simulink library "flatball_6dof_plnt_lib"  (R2021b)
settings: Solver=VariableStepAuto  StartTime=0.0  StopTime=10.0  RelTol=1e-3
values from neighbouring files (symbols this model uses):
  amb = evalin( 'base', 'amb')    [flatball_6dof_eqom.m]
  C = evalin( 'base', 'C')    [flatball_6dof_eqom.m]
  disc = evalin( 'base', 'disc')    [flatball_6dof_eqom.m]    (also in flatball_6dof_init.m = struct; flatball_init_disc_params.m = struct)
  X0_z1m_at_rest = [1e-3 1e-3 -1, -1e-6 1e-6 -1e-6, 0 0 1e-6, 0 0 -1e-6]    [flatball_6dof_wrk.m]    (also in hummel_thesis_mdl_validation.m)
  Y0 = [0 0 -1, 0 15*C.DEG2RAD 0, 15 0 0, 0 0 (2*15*0.29/disc.d)]    [flatball_6dof_eqom.m]
undefined symbols (not defined in the file or in its folder): CandP, flatball
libraries: simulink x6, aerolibanim x2, aerolibnav x2, matrix_library x2, $bdroot x1, mspfiltlib x1
(part 1 of 3)
settings Model: Creator=schae  LastModifiedBy=schae

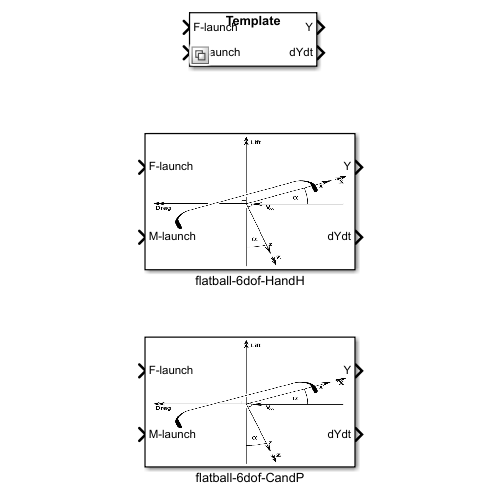
[thumbnail: Simulink's stored preview of the top-level diagram]
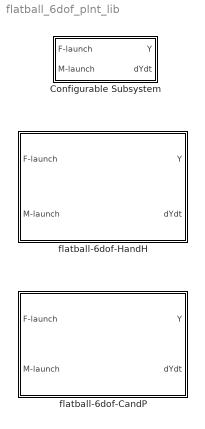
== system flatball_6dof_plnt_lib ==
  Configurable Subsystem : Subsystem  BlockChoice=flatball-6dof-CandP
      settings: TemplateBlock=self  MemberBlocks=flatball-6dof-CandP,flatball-6dof-HandH
  flatball-6dof-CandP : Subsystem
      mask Display: image('C:\.local\desktop\flatball-dev-main-misc.protolabs\media\img\screenshots\flatball-6dof.png'); % Use "Edit Image" on toolstrip to change.
  flatball-6dof-HandH : Subsystem
      mask Display: image('C:\.local\desktop\flatball-dev-main-misc.protolabs\media\img\screenshots\flatball-6dof.png'); % Use "Edit Image" on toolstrip to change.

== system flatball_6dof_plnt_lib/Configurable Subsystem ==
  F-launch : Inport
  M-launch : Inport  Port=2
  flatball-6dof-CandP : $bdroot/flatball-6dof-CandP  SystemSampleTime=-1  VariantActivationTime=update diagram  Latency=0  AutoFrameSizeCalculation=off
  Y : Outport
  dYdt : Outport  Port=2
  wires:
  F-launch/1 -> flatball-6dof-CandP/1
  M-launch/1 -> flatball-6dof-CandP/2
  flatball-6dof-CandP/1 -> Y/1
  flatball-6dof-CandP/2 -> dYdt/1

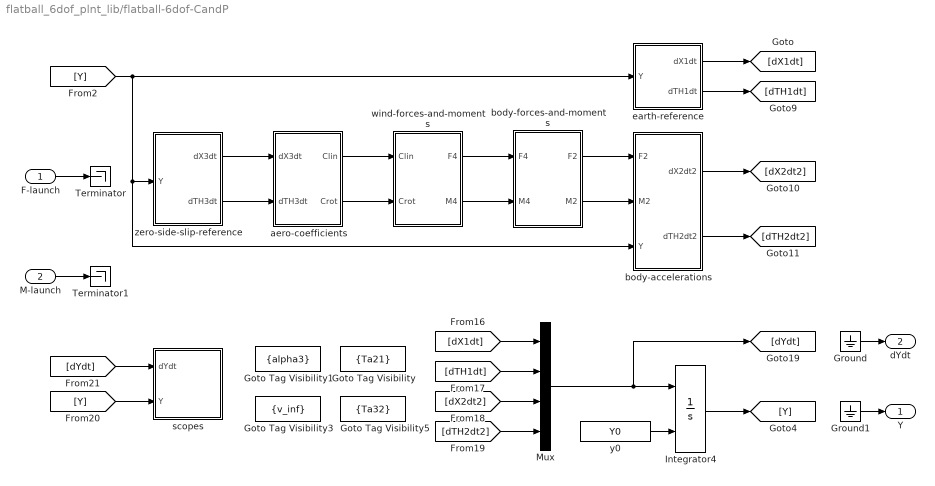
== system flatball_6dof_plnt_lib/flatball-6dof-CandP ==
  F-launch : Inport
  M-launch : Inport  Port=2
  Goto Tag Visibility : GotoTagVisibility  GotoTag=Ta21
  Goto Tag Visibility1 : GotoTagVisibility  GotoTag=alpha3
  Goto Tag Visibility3 : GotoTagVisibility  GotoTag=v_inf
  Goto Tag Visibility5 : GotoTagVisibility  GotoTag=Ta32
  Ground : Ground
  Ground1 : Ground
  Integrator4 : Integrator  InitialConditionSource=external
  Mux : Mux
  Terminator : Terminator
  Terminator1 : Terminator
  aero-coefficients : Subsystem
  body-accelerations : Subsystem
  body-forces-and-moments : Subsystem
  earth-reference : Subsystem
  scopes : Subsystem
  wind-forces-and-moments : Subsystem
  y0 : Constant  Value=Y0
  zero-side-slip-reference : Subsystem
  Y : Outport
  dYdt : Outport  Port=2
  wires:
  y0/1 -> Integrator4/2
  [Y] -> zero-side-slip-reference/1(Y), body-accelerations/3(Y), earth-reference/1(Y)
  zero-side-slip-reference/1(dX3dt) -> aero-coefficients/1(dX3dt)
  [dYdt] -> scopes/1(dYdt)
  Integrator4/1 -> [Y]
  F-launch/1 -> Terminator/1
  [dTH2dt2] -> Mux/4
  body-accelerations/2(dTH2dt2) -> [dTH2dt2]
  earth-reference/2(dTH1dt) -> [dTH1dt]
  earth-reference/1(dX1dt) -> [dX1dt]
  zero-side-slip-reference/2(dTH3dt) -> aero-coefficients/2(dTH3dt)
  body-forces-and-moments/1(F2) -> body-accelerations/1(F2)
  [Y] -> scopes/2(Y)
  [dTH1dt] -> Mux/2
  aero-coefficients/2(Crot) -> wind-forces-and-moments/2(Crot)
  [dX2dt2] -> Mux/3
  body-accelerations/1(dX2dt2) -> [dX2dt2]
  aero-coefficients/1(Clin) -> wind-forces-and-moments/1(Clin)
  [dX1dt] -> Mux/1
  Mux/1 -> [dYdt], Integrator4/1
  wind-forces-and-moments/1(F4) -> body-forces-and-moments/1(F4)
  body-forces-and-moments/2(M2) -> body-accelerations/2(M2)
  wind-forces-and-moments/2(M4) -> body-forces-and-moments/2(M4)
  Ground/1 -> dYdt/1
  M-launch/1 -> Terminator1/1
  Ground1/1 -> Y/1

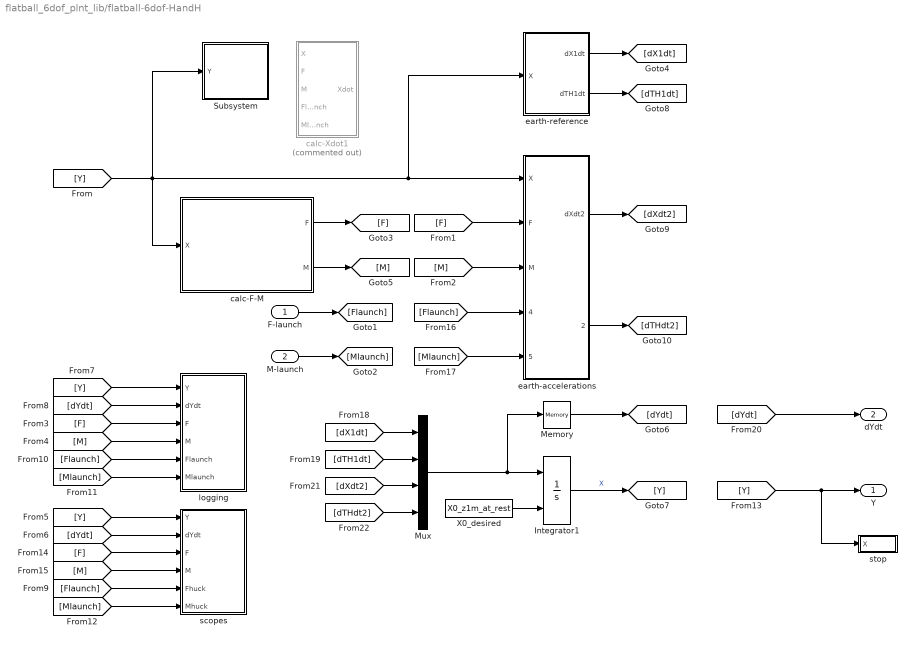
== system flatball_6dof_plnt_lib/flatball-6dof-HandH ==
  F-launch : Inport
  M-launch : Inport  Port=2
  Integrator1 : Integrator  InitialConditionSource=external
  Memory : Memory
  Mux : Mux
  Subsystem : Subsystem
  X0_desired : Constant  Value=X0_z1m_at_rest
  calc-F-M : Subsystem
  calc-Xdot1 : Subsystem  Commented=on
  earth-accelerations : Subsystem
  earth-reference : Subsystem
  logging : Subsystem
  scopes : Subsystem
  stop : Subsystem
  Y : Outport
  dYdt : Outport  Port=2
  wires:
  Mux/1 -> Integrator1/1, Memory/1
  [dX1dt] -> Mux/1
  [dTH1dt] -> Mux/2
  [dXdt2] -> Mux/3
  [dTHdt2] -> Mux/4
  earth-accelerations/2(dTHdt2) -> [dTHdt2]
  earth-accelerations/1(dXdt2) -> [dXdt2]
  earth-reference/2(dTH1dt) -> [dTH1dt]
  earth-reference/1(dX1dt) -> [dX1dt]
  Memory/1 -> [dYdt]
  [Mlaunch] -> earth-accelerations/5(Mlaunch)
  [Flaunch] -> earth-accelerations/4(Flaunch)
  Integrator1/1 -> [Y]  "X"
  calc-F-M/1(F) -> [F]
  calc-F-M/2(M) -> [M]
  [F] -> earth-accelerations/2(F)
  X0_desired/1 -> Integrator1/2
  [M] -> earth-accelerations/3(M)
  [Y] -> calc-F-M/1(X), Subsystem/1(Y), earth-accelerations/1(X), earth-reference/1(X)
  M-launch/1 -> [Mlaunch]
  F-launch/1 -> [Flaunch]
  [dYdt] -> dYdt/1
  [Y] -> Y/1, stop/1(X)
  [Y] -> logging/1(Y)
  [dYdt] -> logging/2(dYdt)
  [dYdt] -> scopes/2(dYdt)
  [Y] -> scopes/1(Y)
  [F] -> logging/3(F)
  [Mlaunch] -> scopes/6(Mhuck)
  [Flaunch] -> logging/5(Flaunch)
  [Mlaunch] -> logging/6(Mlaunch)
  [M] -> logging/4(M)
  [F] -> scopes/3(F)
  [M] -> scopes/4(M)
  [Flaunch] -> scopes/5(Fhuck)

== system flatball_6dof_plnt_lib/flatball-6dof-CandP/aero-coefficients ==
  dX3dt : Inport
  dTH3dt : Inport  Port=2
  Mux1 : Mux  Inputs=3
  Mux2 : Mux  Inputs=3
  Subsystem : Subsystem
  Subsystem1 : Subsystem
  Subsystem2 : Subsystem
  Subsystem3 : Subsystem
  Subsystem4 : Subsystem
  Subsystem5 : Subsystem
  alpha3 : Subsystem
  Clin : Outport
  Crot : Outport  Port=2
  wires:
  Subsystem4/1(CN) -> Mux1/3  "CN"
  Subsystem3/1(CL) -> Mux1/1  "CL"
  [v_inf] -> Subsystem4/2(v_inf), Subsystem2/3(v_inf), Subsystem3/2(v_inf), Subsystem5/2(v_inf)
  Subsystem2/1(CM) -> Mux1/2  "CM"
  Subsystem1/1(Clift) -> Mux2/3  "Clift"
  Subsystem/1(Cdrag) -> Mux2/1  "Cdrag"
  Subsystem5/1(Cside) -> Mux2/2  "Cside"
  [alpha3] -> Subsystem1/1(alpha3), Subsystem2/2(alpha3), Subsystem/1(alpha3)
  alpha3/1(alpha3) -> [alpha3]
  Mux1/1 -> Crot/1
  dTH3dt/1 -> Subsystem5/1(dTH3dt), Subsystem4/1(dTH3dt), Subsystem2/1(dTH3dt), Subsystem3/1(dTH3dt)
  Mux2/1 -> Clin/1
  dX3dt/1 -> alpha3/1(dX3dt)

== system flatball_6dof_plnt_lib/flatball-6dof-CandP/body-accelerations ==
  F2 : Inport
  M2 : Inport  Port=2
  Y : Inport  Port=3
  Product{,2..4} (4 alike) : Product  Multiplication=Matrix(*)
  Product1 : Product  Inputs=**
  Sum : Sum  Inputs=+-
  Sum1 : Sum  Inputs=+-
  dTH2dt : Selector  InputPortWidth=12  IndexOptions=Index vector (dialog)  Indices=[10 11 12]  OutputSizes=1
  dX2dt : Selector  InputPortWidth=12  IndexOptions=Index vector (dialog)  Indices=[7 8 9]  OutputSizes=1
  mg : Constant  Value=disc.m ^ -1
  mg1 : Constant  Value=disc.I ^ -1
  mg2 : Constant  Value=disc.I
  w-tilde : MATLAB Function  TreatAsAtomicUnit=on
  dX2dt2 : Outport
  dTH2dt2 : Outport  Port=2
  wires:
  Sum1/1 -> Product4/2
  Product3/1 -> Sum1/2
  [w] -> Product2/1
  mg1/1 -> Product4/1
  [dTH2dt] -> Product3/2
  [dTH2dt] -> w-tilde/1(dTH2dt)
  dTH2dt/1 -> [dTH2dt]
  Product2/1 -> Product3/1
  mg2/1 -> Product2/2
  [w] -> Product/1
  w-tilde/1(w) -> [w]
  Product/1 -> Sum/2
  Product1/1 -> Sum/1
  mg/1 -> Product1/2
  F2/1 -> Product1/1
  dX2dt/1 -> Product/2
  Product4/1 -> dTH2dt2/1  "dTH2dt2"
  M2/1 -> Sum1/1
  Sum/1 -> dX2dt2/1  "dX2dt2"
  Y/1 -> dX2dt/1, dTH2dt/1

== system flatball_6dof_plnt_lib/flatball-6dof-CandP/body-forces-and-moments ==
  F4 : Inport
  M4 : Inport  Port=2
  Ground : Ground
  Ground1 : Ground
  Mux : Mux  Inputs=3
  Product{,1..3} (4 alike) : Product  Multiplication=Matrix(*)
  Product4 : Product
  Sum : Sum  Inputs=2
  Transpose1 : Math  Operator=transpose  SaturateOnIntegerOverflow=on
  Transpose2 : Math  Operator=transpose  SaturateOnIntegerOverflow=on
  attitude-transform : MATLAB Function  TreatAsAtomicUnit=on
  mg : Constant  Value=disc.m * amb.g
  mg1 : Constant  Value=[0 0 1]'
  F2 : Outport
  M2 : Outport  Port=2
  wires:
  M4/1 -> Product1/2
  Transpose1/1 -> Product3/1  "Ta12"
  mg1/1 -> Product4/2
  mg/1 -> Product4/1
  Transpose2/1 -> Product2/2  "Ta43"
  Product4/1 -> Product3/2
  Product3/1 -> Sum/2  "F2g"
  Sum/1 -> F2/1  "F2"
  [Ta42] -> Product1/1
  [Ta42] -> Product/1
  Product2/1 -> [Ta42]
  [Ta34] -> Transpose2/1
  [Ta32] -> Product2/1
  attitude-transform/1(T) -> [Ta34]
  Ground/1 -> Mux/3
  Mux/1 -> attitude-transform/1(TH)
  Ground1/1 -> Mux/1
  Product1/1 -> M2/1  "M2"
  [Ta21] -> Transpose1/1
  Product/1 -> Sum/1  "F2aero"
  F4/1 -> Product/2
  [alpha3] -> Mux/2

== system flatball_6dof_plnt_lib/flatball-6dof-CandP/earth-reference ==
  Y : Inport
  Product : Product  Multiplication=Matrix(*)
  Product1 : Product  Multiplication=Matrix(*)
  TH1 : Selector  InputPortWidth=12  IndexOptions=Index vector (dialog)  Indices=[4 5 6]  OutputSizes=1
  Terminator : Terminator
  X1 : Selector  InputPortWidth=12  IndexOptions=Index vector (dialog)  Indices=[1 2 3]  OutputSizes=1
  attitude-transform : MATLAB Function  TreatAsAtomicUnit=on
  dTH2dt : Selector  InputPortWidth=12  IndexOptions=Index vector (dialog)  Indices=[10 11 12]  OutputSizes=1
  dX2dt : Selector  InputPortWidth=12  IndexOptions=Index vector (dialog)  Indices=[7 8 9]  OutputSizes=1
  logs : Subsystem
  rate-transform : MATLAB Function  TreatAsAtomicUnit=on
  v_inf : Subsystem
  dX1dt : Outport
  dTH1dt : Outport  Port=2
  tag scope: Ta21=scoped
  wires:
  dTH2dt/1 -> Product1/2
  [Tr21] -> Product1/1
  [Ta21] -> Product/1
  rate-transform/1(T) -> [Tr21]
  attitude-transform/1(T) -> [Ta21]
  X1/1 -> Terminator/1  "X1"
  Product1/1 -> dTH1dt/1  "TH1dot"
  Product/1 -> dX1dt/1  "X1dot"
  TH1/1 -> attitude-transform/1(TH), rate-transform/1(TH)  "TH1"
  dX2dt/1 -> Product/2, v_inf/1(dX2dt)
  Y/1 -> TH1/1, dX2dt/1, dTH2dt/1, logs/1(Y), X1/1

== system flatball_6dof_plnt_lib/flatball-6dof-CandP/scopes ==
  dYdt : Inport
  Y : Inport  Port=2
  Compare To Constant : simulink/Logic and Bit Operations/Compare To Constant  relop=>=  const=0.0  OutDataTypeStr=boolean
  Demux : Demux  Outputs=[3 3 3 3]
  Demux1 : Demux  Outputs=[3 3 3 3]
  Selector : Selector  InputPortWidth=3  IndexOptions=Index vector (dialog)  Indices=[3]  OutputSizes=1
  Selector1 : Selector  InputPortWidth=3  IndexOptions=Index vector (dialog)  Indices=[1 2]  OutputSizes=1
  Stop Simulation : Stop
  TH1 : Scope
  X1 : Scope
  dTH1dt : Scope
  dTH2dt : Scope
  dTH2dt2 : Scope
  dX1dt : Scope
  dX2dt : Scope
  dX2dt2 : Scope
  wires:
  Demux1/3 -> dX2dt2/1
  Demux1/4 -> dTH2dt2/1
  Demux1/2 -> dTH1dt/1
  Demux1/1 -> dX1dt/1
  dYdt/1 -> Demux1/1
  Demux/4 -> dTH2dt/1
  Demux/3 -> dX2dt/1
  Demux/2 -> Selector1/1
  Demux/1 -> X1/1, Selector/1
  Y/1 -> Demux/1
  Selector1/1 -> TH1/1
  Selector/1 -> Compare To Constant/1
  Compare To Constant/1 -> Stop Simulation/1

== system flatball_6dof_plnt_lib/flatball-6dof-CandP/wind-forces-and-moments ==
  Clin : Inport
  Crot : Inport  Port=2
  Demux : Demux  Outputs=3
  Demux1 : Demux  Outputs=3
  Gain{,1..3} (4 alike) : Gain  Gain=-1
  Gain4 : Gain  Gain=0
  Mux : Mux  Inputs=3
  Product : Product
  Product1 : Product
  Subsystem : Subsystem
  Terminator : Terminator
  Terminator1 : Terminator
  Terminator2 : Terminator
  F4 : Outport
  M4 : Outport  Port=2
  wires:
  [v_inf] -> Subsystem/1(v_inf)
  Crot/1 -> Product1/2
  Subsystem/2(qSc) -> Product1/1
  Subsystem/1(qS) -> Product/2
  Mux/1 -> Product/1
  Gain2/1 -> Mux/1
  Gain4/1 -> Mux/2
  Gain3/1 -> Mux/3
  Demux1/1 -> Gain2/1
  Demux1/2 -> Gain4/1
  Clin/1 -> Demux1/1
  Demux1/3 -> Gain3/1
  Gain/1 -> Terminator/1  "drag"
  Gain1/1 -> Terminator2/1  "lift"
  [F4] -> Demux/1
  Demux/3 -> Gain1/1
  Demux/1 -> Gain/1
  Demux/2 -> Terminator1/1
  Product1/1 -> M4/1  "M4"
  Product/1 -> F4/1, [F4]  "F4"

== system flatball_6dof_plnt_lib/flatball-6dof-CandP/zero-side-slip-reference ==
  Y : Inport
  Ground : Ground
  Ground1 : Ground
  Mux : Mux  Inputs=3
  Product : Product  Multiplication=Matrix(*)
  Product1 : Product  Multiplication=Matrix(*)
  Transpose : Math  Operator=transpose  SaturateOnIntegerOverflow=on
  attitude-transform : MATLAB Function  TreatAsAtomicUnit=on
  beta2 : Subsystem
  dTH2dt : Selector  InputPortWidth=12  IndexOptions=Index vector (dialog)  Indices=[10 11 12]  OutputSizes=1
  dX2dt : Selector  InputPortWidth=12  IndexOptions=Index vector (dialog)  Indices=[7 8 9]  OutputSizes=1
  dX3dt : Outport
  dTH3dt : Outport  Port=2
  tag scope: Ta32=scoped
  wires:
  Transpose/1 -> [Ta23]  "Ta23"
  [Ta32] -> Transpose/1
  [Ta23] -> Product/1, Product1/1
  attitude-transform/1(T) -> [Ta32]
  Ground1/1 -> Mux/1
  Ground/1 -> Mux/2
  Mux/1 -> attitude-transform/1(TH)
  beta2/1(beta2) -> Mux/3
  dTH2dt/1 -> Product1/2  "dTH2dt"
  dX2dt/1 -> Product/2, beta2/1(dX2dt)  "dX2dt"
  Product/1 -> dX3dt/1  "dX3dt"
  Product1/1 -> dTH3dt/1  "dTH3dt"
  Y/1 -> dTH2dt/1, dX2dt/1

== system flatball_6dof_plnt_lib/flatball-6dof-HandH/Subsystem ==
  Y : Inport
  Product : Product  Multiplication=Matrix(*)
  Scope : Scope  NumInputPorts=2
  TH : Selector  InputPortWidth=12  IndexOptions=Index vector (dialog)  Indices=[4 5 6]  OutputSizes=1
  TH1 : Selector  InputPortWidth=3  IndexOptions=Index vector (dialog)  Indices=[1 2]  OutputSizes=1
  TH2 : Selector  InputPortWidth=3  IndexOptions=Index vector (dialog)  Indices=[1 2]  OutputSizes=1
  Terminator : Terminator
  Transpose : Math  Operator=transpose  SaturateOnIntegerOverflow=on
  attitude-transform : MATLAB Function  TreatAsAtomicUnit=on
  rate-transform : MATLAB Function  TreatAsAtomicUnit=on
  wires:
  TH2/1 -> Scope/2
  TH1/1 -> Scope/1
  Product/1 -> TH2/1  "TH2"
  Transpose/1 -> Product/1
  [Ta21] -> Transpose/1
  [Tr21] -> Terminator/1
  Y/1 -> TH/1
  attitude-transform/1(T) -> [Ta21]
  rate-transform/1(T) -> [Tr21]
  TH/1 -> attitude-transform/1(TH), rate-transform/1(TH), TH1/1, Product/2

== system flatball_6dof_plnt_lib/flatball-6dof-HandH/calc-F-M ==
  X : Inport
  From1 : From  Commented=on  GotoTag=X
  From10 : From  Commented=on  GotoTag=F
  From11 : From  Commented=on  GotoTag=M
  From5 : From  Commented=on  GotoTag=alpha
  From6 : From  Commented=on  GotoTag=T
  From9 : From  Commented=on  GotoTag=wD
  TH : Selector  InputPortWidth=12  IndexOptions=Index vector (dialog)  Indices=[4 5 6]  OutputSizes=1
  T_c_N : MATLAB Function  TreatAsAtomicUnit=on
  calc-F : Subsystem
  calc-M : Subsystem
  calc-alpha : Subsystem
  lab : Subsystem  Commented=on
  F : Outport
  M : Outport  Port=2
  wires:
  T_c_N/1(T_c_N) -> [T]
  TH/1 -> T_c_N/1(TH)
  calc-M/1(M) -> M/1  "M2"
  calc-F/1(F) -> F/1  "F2"
  From5/1 -> lab/4(alpha)
  calc-alpha/1(alpha) -> [alpha]
  From11/1 -> lab/6(M)
  [alpha] -> calc-M/3(alpha), calc-F/3(alpha)
  [T] -> calc-alpha/2(T_c_N)
  From9/1 -> lab/3(wD)
  [T] -> calc-F/2(T_c_N), calc-M/2(T_c_N)
  X/1 -> calc-F/1(X), calc-alpha/1(X), calc-M/1(X), TH/1
  From6/1 -> lab/2(T)
  From10/1 -> lab/5(F)
  From1/1 -> lab/1(X)

== system flatball_6dof_plnt_lib/flatball-6dof-HandH/calc-Xdot1 ==
  X : Inport
  F : Inport  Port=2
  M : Inport  Port=3
  Flaunch : Inport  Port=4
  Mlaunch : Inport  Port=5
  Mux{,1..3} (4 alike) : Mux  Inputs=2
  Product1 : Product  Inputs=*/
  Reshape : Reshape
  Reshape1 : Reshape
  Reshape2 : Reshape
  Scope : Scope
  Scope1 : Scope
  Scope2 : Scope
  Selector : Selector  InputPortWidth=12  IndexOptions=Index vector (dialog)  Indices=[1 2 3 7 8 9 4 5 6 10 11 12]  OutputSizes=1
  Sum : Sum  Inputs=2
  calc-THdot : MATLAB Function  TreatAsAtomicUnit=on
  calc-Xdot : MATLAB Function  TreatAsAtomicUnit=on
  dTHdt : Selector  InputPortWidth=12  IndexOptions=Index vector (dialog)  Indices=[10 11 12]  OutputSizes=1
  dXdt : Selector  InputPortWidth=12  IndexOptions=Index vector (dialog)  Indices=[7 8 9]  OutputSizes=1
  mg : Constant  Value=disc.m
  Xdot : Outport
  wires:
  Mux/1 -> Selector/1
  X/1 -> dTHdt/1, dXdt/1, calc-THdot/1(X)
  M/1 -> calc-THdot/2(M)
  Selector/1 -> Xdot/1
  Mlaunch/1 -> calc-THdot/3(Mlaunch)
  F/1 -> Reshape2/1, calc-Xdot/2(F)
  Flaunch/1 -> calc-Xdot/3(Flaunch), Sum/2
  mg/1 -> Product1/2
  Sum/1 -> Scope2/1, Product1/1
  Product1/1 -> Mux1/2
  calc-THdot/1(dTHdt2) -> Reshape1/1  "THdot"
  calc-Xdot/1(Xdot) -> Reshape/1  "Xdot"
  Mux1/1 -> Mux/1, Scope/1
  Reshape2/1 -> Sum/1
  dXdt/1 -> Mux3/1, calc-Xdot/1(dXdt), Mux1/1
  dTHdt/1 -> Mux2/1
  Reshape1/1 -> Mux2/2
  Mux2/1 -> Mux/2
  Reshape/1 -> Mux3/2

== system flatball_6dof_plnt_lib/flatball-6dof-HandH/earth-accelerations ==
  X : Inport
  F : Inport  Port=2
  M : Inport  Port=3
  Flaunch : Inport  Port=4
  Mlaunch : Inport  Port=5
  Product1 : Product  Inputs=*/
  Sum : Sum  Inputs=2
  Sum1 : Sum  Inputs=2
  calc-THdot : MATLAB Function  TreatAsAtomicUnit=on
  mg : Constant  Value=disc.m
  dXdt2 : Outport
  dTHdt2 : Outport  Port=2
  wires:
  Sum1/1 -> calc-THdot/2(M)
  M/1 -> Sum1/1
  Mlaunch/1 -> Sum1/2
  F/1 -> Sum/1
  calc-THdot/1(dTHdt2) -> dTHdt2/1  "THdot"
  Product1/1 -> dXdt2/1
  Sum/1 -> Product1/1
  mg/1 -> Product1/2
  Flaunch/1 -> Sum/2
  X/1 -> calc-THdot/1(X)

== system flatball_6dof_plnt_lib/flatball-6dof-HandH/earth-reference ==
  X : Inport
  dTHdt : Selector  InputPortWidth=12  IndexOptions=Index vector (dialog)  Indices=[10 11 12]  OutputSizes=1
  dXdt : Selector  InputPortWidth=12  IndexOptions=Index vector (dialog)  Indices=[7 8 9]  OutputSizes=1
  dX1dt : Outport
  dTH1dt : Outport  Port=2
  wires:
  dXdt/1 -> dX1dt/1
  dTHdt/1 -> dTH1dt/1
  X/1 -> dTHdt/1, dXdt/1

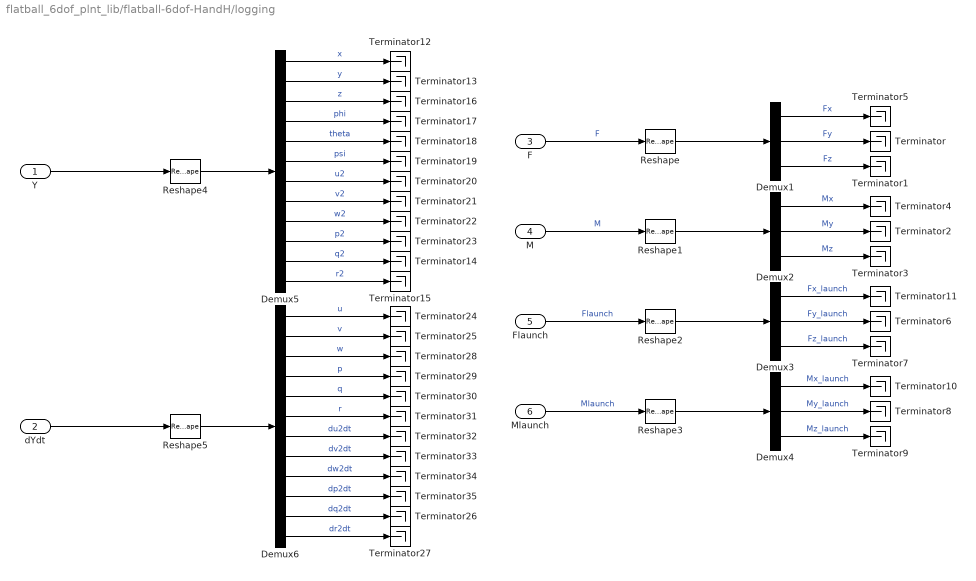
== system flatball_6dof_plnt_lib/flatball-6dof-HandH/logging ==
  Y : Inport
  dYdt : Inport  Port=2
  F : Inport  Port=3
  M : Inport  Port=4
  Flaunch : Inport  Port=5
  Mlaunch : Inport  Port=6
  Demux{1..4} (4 alike) : Demux  Outputs=3
  Demux5 : Demux  Outputs=[1 1 1 1 1 1 1 1 1 1 1 1]
  Demux6 : Demux  Outputs=[1 1 1 1 1 1 1 1 1 1 1 1]
  Reshape{,1..5} (6 alike) : Reshape
  Terminator{,1..35} (36 alike) : Terminator
  wires:
  Demux6/3 -> Terminator28/1  "w"
  Demux6/1 -> Terminator24/1  "u"
  Demux6/8 -> Terminator33/1  "dv2dt"
  Demux6/9 -> Terminator34/1  "dw2dt"
  Reshape5/1 -> Demux6/1
  Demux6/2 -> Terminator25/1  "v"
  Demux6/12 -> Terminator27/1  "dr2dt"
  Demux6/10 -> Terminator35/1  "dp2dt"
  Demux6/7 -> Terminator32/1  "du2dt"
  Demux6/5 -> Terminator30/1  "q"
  Demux6/6 -> Terminator31/1  "r"
  Demux6/11 -> Terminator26/1  "dq2dt"
  Demux6/4 -> Terminator29/1  "p"
  dYdt/1 -> Reshape5/1
  Y/1 -> Reshape4/1
  Demux5/4 -> Terminator17/1  "phi"
  Demux5/11 -> Terminator14/1  "q2"
  Demux5/6 -> Terminator19/1  "psi"
  Demux5/5 -> Terminator18/1  "theta"
  Demux5/7 -> Terminator20/1  "u2"
  Demux5/10 -> Terminator23/1  "p2"
  Demux5/12 -> Terminator15/1  "r2"
  Demux5/2 -> Terminator13/1  "y"
  Reshape4/1 -> Demux5/1
  Demux5/9 -> Terminator22/1  "w2"
  Demux5/8 -> Terminator21/1  "v2"
  Demux5/1 -> Terminator12/1  "x"
  Demux5/3 -> Terminator16/1  "z"
  Mlaunch/1 -> Reshape3/1  "Mlaunch"
  F/1 -> Reshape/1  "F"
  Demux3/2 -> Terminator6/1  "Fy_launch"
  Demux3/1 -> Terminator11/1  "Fx_launch"
  Flaunch/1 -> Reshape2/1  "Flaunch"
  Reshape3/1 -> Demux4/1
  Demux4/3 -> Terminator9/1  "Mz_launch"
  Demux4/1 -> Terminator10/1  "Mx_launch"
  Reshape/1 -> Demux1/1
  Demux1/1 -> Terminator5/1  "Fx"
  Demux4/2 -> Terminator8/1  "My_launch"
  M/1 -> Reshape1/1  "M"
  Demux3/3 -> Terminator7/1  "Fz_launch"
  Demux2/2 -> Terminator2/1  "My"
  Demux1/2 -> Terminator/1  "Fy"
  Demux1/3 -> Terminator1/1  "Fz"
  Reshape2/1 -> Demux3/1
  Demux2/1 -> Terminator4/1  "Mx"
  Demux2/3 -> Terminator3/1  "Mz"
  Reshape1/1 -> Demux2/1

== system flatball_6dof_plnt_lib/flatball-6dof-HandH/scopes ==
  Y : Inport
  dYdt : Inport  Port=2
  F : Inport  Port=3
  M : Inport  Port=4
  Fhuck : Inport  Port=5
  Mhuck : Inport  Port=6
  Compare To Constant : simulink/Logic and Bit Operations/Compare To Constant  relop=>=  const=0.0  OutDataTypeStr=boolean
  Demux : Demux  Outputs=[3 3 3 3]
  Demux1 : Demux  Outputs=[3 3 3 3]
  Selector : Selector  InputPortWidth=3  IndexOptions=Index vector (dialog)  Indices=[3]  OutputSizes=1
  Selector1 : Selector  InputPortWidth=3  IndexOptions=Index vector (dialog)  Indices=[1 2]  OutputSizes=1
  Stop Simulation : Stop
  Sum1 : Sum
  Sum2 : Sum
  TH1 : Scope
  TH1dot : Scope
  TH2dot : Scope
  TH2dotdot : Scope
  X1 : Scope
  X1dot : Scope
  X2dot : Scope
  X2dotdot : Scope
  eml-6dof : Subsystem  Commented=on
  flatball-F,M : Scope  NumInputPorts=2
  huck-F,M : Scope  NumInputPorts=2
  net-F,M : Scope  NumInputPorts=2
  work-in-progress : Subsystem  Commented=on
  wires:
  Demux/1 -> Selector/1, X1/1
  Demux1/3 -> X2dotdot/1
  Y/1 -> Demux/1
  Compare To Constant/1 -> Stop Simulation/1
  Demux1/4 -> TH2dotdot/1
  Demux/3 -> X2dot/1
  Demux1/1 -> X1dot/1
  Selector1/1 -> TH1/1
  Demux/2 -> Selector1/1
  Demux1/2 -> TH1dot/1
  Selector/1 -> Compare To Constant/1
  dYdt/1 -> Demux1/1
  Demux/4 -> TH2dot/1
  M/1 -> flatball-F,M/2, Sum2/1
  F/1 -> flatball-F,M/1, Sum1/1
  Fhuck/1 -> huck-F,M/1, Sum1/2
  Sum1/1 -> net-F,M/1
  Mhuck/1 -> huck-F,M/2, Sum2/2
  Sum2/1 -> net-F,M/2

== system flatball_6dof_plnt_lib/flatball-6dof-HandH/stop ==
  X : Inport
  Compare To Constant : simulink/Logic and Bit Operations/Compare To Constant  relop=>=  const=0  OutDataTypeStr=boolean
  Selector : Selector  InputPortWidth=12  IndexOptions=Index vector (dialog)  Indices=[3]  OutputSizes=1
  Stop Simulation : Stop
  wires:
  X/1 -> Selector/1
  Compare To Constant/1 -> Stop Simulation/1
  Selector/1 -> Compare To Constant/1

== system flatball_6dof_plnt_lib/flatball-6dof-CandP/aero-coefficients/Subsystem ==
  alpha3 : Inport
  1-D Lookup Table : Lookup_n-D  NumberOfTableDimensions=1  BreakpointsForDimension1=disc.aoa_data  Table=disc.Cdrag_data  InterpMethod=Cubic spline  ExtrapMethod=Cubic spline  InternalRulePriority=Speed  RndMeth=Simplest  InputSameDT=on
  Math Function : Math  Operator=square  SaturateOnIntegerOverflow=on
  Product1 : Product  Inputs=**
  Sum1 : Sum
  Sum2 : Sum  Inputs=+-
  Terminator : Terminator
  mg : Constant  Value=disc.CD0
  mg1 : Constant  Value=disc.CDa
  mg2 : Constant  Value=disc.alpha0
  Cdrag : Outport
  wires:
  Sum1/1 -> Terminator/1
  1-D Lookup Table/1 -> Cdrag/1
  Math Function/1 -> Product1/2
  mg2/1 -> Sum2/2
  Sum2/1 -> Math Function/1
  Product1/1 -> Sum1/2
  mg/1 -> Sum1/1
  mg1/1 -> Product1/1
  alpha3/1 -> Sum2/1, 1-D Lookup Table/1

== system flatball_6dof_plnt_lib/flatball-6dof-CandP/aero-coefficients/Subsystem1 ==
  alpha3 : Inport
  1-D Lookup Table : Lookup_n-D  NumberOfTableDimensions=1  BreakpointsForDimension1=disc.aoa_data  Table=disc.Clift_data  InterpMethod=Cubic spline  ExtrapMethod=Cubic spline  InternalRulePriority=Speed  RndMeth=Simplest  InputSameDT=on
  Product1 : Product  Inputs=**
  Sum1 : Sum
  Terminator : Terminator
  mg : Constant  Value=disc.CL0
  mg1 : Constant  Value=disc.CLa
  Clift : Outport
  wires:
  Sum1/1 -> Terminator/1
  1-D Lookup Table/1 -> Clift/1
  alpha3/1 -> Product1/2, 1-D Lookup Table/1
  mg1/1 -> Product1/1
  mg/1 -> Sum1/1
  Product1/1 -> Sum1/2

== system flatball_6dof_plnt_lib/flatball-6dof-CandP/aero-coefficients/Subsystem2 ==
  dTH3dt : Inport
  alpha3 : Inport  Port=2
  v_inf : Inport  Port=3
  1-D Lookup Table : Lookup_n-D  NumberOfTableDimensions=1  BreakpointsForDimension1=disc.aoa_data  Table=disc.CM_data  InterpMethod=Cubic spline  ExtrapMethod=Cubic spline  InternalRulePriority=Speed  RndMeth=Simplest  InputSameDT=on
  Gain : Gain  Gain=2
  Product1 : Product  Inputs=**
  Product2 : Product  Inputs=*/
  Product3 : Product  Inputs=**
  Product4 : Product  Inputs=**
  Selector : Selector  InputPortWidth=3  IndexOptions=Index vector (dialog)  Indices=[2]  OutputSizes=1
  Sum1 : Sum
  Sum2 : Sum
  Terminator : Terminator
  mg : Constant  Value=disc.CM0
  mg1 : Constant  Value=disc.CMa
  mg2 : Constant  Value=disc.c
  mg3 : Constant  Value=disc.CMq
  CM : Outport
  wires:
  Sum1/1 -> CM/1
  Product4/1 -> Sum1/2
  Sum2/1 -> Terminator/1
  mg/1 -> Sum2/1
  1-D Lookup Table/1 -> Sum1/1
  Product1/1 -> Sum2/2
  Selector/1 -> Product3/1  "q3"
  mg3/1 -> Product4/1
  Product3/1 -> Product4/2
  Product2/1 -> Product3/2
  dTH3dt/1 -> Selector/1
  alpha3/1 -> Product1/1, 1-D Lookup Table/1
  mg1/1 -> Product1/2
  v_inf/1 -> Gain/1
  Gain/1 -> Product2/2
  mg2/1 -> Product2/1

== system flatball_6dof_plnt_lib/flatball-6dof-CandP/aero-coefficients/Subsystem3 ==
  dTH3dt : Inport
  v_inf : Inport  Port=2
  Gain : Gain  Gain=2
  Product1 : Product  Inputs=**
  Product2 : Product  Inputs=*/
  Product3 : Product  Inputs=**
  Selector : Selector  InputPortWidth=3  IndexOptions=Index vector (dialog)  Indices=[1]  OutputSizes=1
  mg1 : Constant  Value=disc.CLp
  mg2 : Constant  Value=disc.c
  CL : Outport
  wires:
  Selector/1 -> Product1/2  "p3"
  Gain/1 -> Product2/2
  Product2/1 -> Product3/2
  Product1/1 -> Product3/1
  dTH3dt/1 -> Selector/1
  mg2/1 -> Product2/1
  v_inf/1 -> Gain/1
  mg1/1 -> Product1/1
  Product3/1 -> CL/1

== system flatball_6dof_plnt_lib/flatball-6dof-CandP/aero-coefficients/Subsystem4 ==
  dTH3dt : Inport
  v_inf : Inport  Port=2
  Gain : Gain  Gain=2
  Product2 : Product  Inputs=*/
  Product3 : Product  Inputs=**
  Product4 : Product  Inputs=**
  Selector : Selector  InputPortWidth=3  IndexOptions=Index vector (dialog)  Indices=[3]  OutputSizes=1
  mg2 : Constant  Value=disc.c
  mg3 : Constant  Value=disc.CNr
  CN : Outport
  wires:
  Selector/1 -> Product3/1  "r3"
  Product4/1 -> CN/1
  mg2/1 -> Product2/1
  Gain/1 -> Product2/2
  v_inf/1 -> Gain/1
  dTH3dt/1 -> Selector/1
  Product2/1 -> Product3/2
  Product3/1 -> Product4/2
  mg3/1 -> Product4/1

== system flatball_6dof_plnt_lib/flatball-6dof-CandP/aero-coefficients/Subsystem5 ==
  dTH3dt : Inport
  v_inf : Inport  Port=2
  Ground : Ground
  Terminator : Terminator
  Terminator1 : Terminator
  Cside : Outport
  wires:
  v_inf/1 -> Terminator1/1
  Ground/1 -> Cside/1
  dTH3dt/1 -> Terminator/1

== system flatball_6dof_plnt_lib/flatball-6dof-CandP/aero-coefficients/alpha3 ==
  dX3dt : Inport
  Atan2 : Trigonometry  Operator=atan2
  Selector : Selector  InputPortWidth=3  IndexOptions=Index vector (dialog)  Indices=[3]  OutputSizes=1
  Selector3 : Selector  InputPortWidth=3  IndexOptions=Index vector (dialog)  Indices=[1]  OutputSizes=1
  alpha3 : Outport
  tag scope: alpha3=scoped
  wires:
  Atan2/1 -> [alpha3], alpha3/1  "alpha"
  Selector/1 -> Atan2/1  "w3"
  Selector3/1 -> Atan2/2  "u3"
  dX3dt/1 -> Selector3/1, Selector/1

== system flatball_6dof_plnt_lib/flatball-6dof-CandP/earth-reference/logs ==
  Y : Inport
  Demux2 : Demux  Outputs=[1 1 1 1 1 1 1 1 1 1 1 1]
  Reshape : Reshape
  Terminator{1..12} (12 alike) : Terminator
  wires:
  Demux2/9 -> Terminator9/1  "w"
  Demux2/6 -> Terminator6/1  "psi"
  Y/1 -> Reshape/1
  Demux2/1 -> Terminator1/1  "x"
  Demux2/3 -> Terminator3/1  "z"
  Demux2/7 -> Terminator7/1  "u"
  Demux2/10 -> Terminator12/1  "p"
  Reshape/1 -> Demux2/1
  Demux2/11 -> Terminator10/1  "q"
  Demux2/8 -> Terminator8/1  "v"
  Demux2/4 -> Terminator4/1  "phi"
  Demux2/2 -> Terminator2/1  "y"
  Demux2/5 -> Terminator5/1  "theta"
  Demux2/12 -> Terminator11/1  "r"

== system flatball_6dof_plnt_lib/flatball-6dof-CandP/earth-reference/v_inf ==
  dX2dt : Inport
  Sqrt : Sqrt  SaturateOnIntegerOverflow=on
  Square3 : Math  Operator=square  SaturateOnIntegerOverflow=on
  Sum1 : Sum  Inputs=1
  tag scope: v_inf=scoped
  wires:
  Sum1/1 -> Sqrt/1
  Square3/1 -> Sum1/1
  dX2dt/1 -> Square3/1
  Sqrt/1 -> [v_inf]  "v_inf"

== system flatball_6dof_plnt_lib/flatball-6dof-CandP/wind-forces-and-moments/Subsystem ==
  v_inf : Inport
  Gain2 : Gain  Gain=0.5
  Math Function : Math  Operator=square  SaturateOnIntegerOverflow=on
  Product : Product
  Product1 : Product
  Product2 : Product
  S : Constant  Value=disc.S
  c : Constant  Value=disc.c
  rho : Constant  Value=amb.rho
  qS : Outport
  qSc : Outport  Port=2
  wires:
  S/1 -> Product1/2
  c/1 -> Product2/2
  Product2/1 -> qSc/1
  Product1/1 -> qS/1, Product2/1
  Product/1 -> Product1/1  "q_inf"
  v_inf/1 -> Math Function/1
  Math Function/1 -> Product/1
  Gain2/1 -> Product/2
  rho/1 -> Gain2/1

== system flatball_6dof_plnt_lib/flatball-6dof-CandP/zero-side-slip-reference/beta2 ==
  dX2dt : Inport
  Atan2 : Trigonometry  Operator=atan2
  Goto3 : Goto  Commented=on  GotoTag=beta2  TagVisibility=scoped
  Selector : Selector  InputPortWidth=3  IndexOptions=Index vector (dialog)  Indices=[2]  OutputSizes=1
  Selector3 : Selector  InputPortWidth=3  IndexOptions=Index vector (dialog)  Indices=[1]  OutputSizes=1
  beta2 : Outport
  wires:
  Atan2/1 -> Goto3/1, beta2/1  "beta"
  Selector/1 -> Atan2/1  "v2"
  Selector3/1 -> Atan2/2  "u2"
  dX2dt/1 -> Selector3/1, Selector/1

== system flatball_6dof_plnt_lib/flatball-6dof-HandH/calc-F-M/calc-F ==
  X : Inport
  T_c_N : Inport  Port=2
  alpha : Inport  Port=3
  Fg_N : Constant  Value=[0 0 disc.m*amb.g]'
  Terminator{,1..3} (4 alike) : Terminator
  aero-coeff : Subsystem
  calc-F : MATLAB Function  TreatAsAtomicUnit=on
  dXdt : Selector  InputPortWidth=12  IndexOptions=Index vector (dialog)  Indices=[7 8 9]  OutputSizes=1
  q-inf : Subsystem
  F : Outport
  wires:
  calc-F/4(vmag) -> Terminator3/1  "v_inf"
  calc-F/3(drag) -> Terminator2/1  "drag"
  calc-F/2(lift) -> Terminator1/1  "lift"
  q-inf/2(q-inf-S-d) -> Terminator/1
  aero-coeff/2(Cd) -> calc-F/5(CDrag)
  aero-coeff/1(Cl) -> calc-F/4(CLift)
  alpha/1 -> aero-coeff/1(alpha)
  q-inf/1(q-inf-S) -> calc-F/6(q_inf_times_S)
  calc-F/1(F) -> F/1  "F"
  Fg_N/1 -> calc-F/3(Fg_N)
  T_c_N/1 -> calc-F/2(T_c_N)
  X/1 -> q-inf/1(X), dXdt/1
  dXdt/1 -> calc-F/1(vel)

== system flatball_6dof_plnt_lib/flatball-6dof-HandH/calc-F-M/calc-M ==
  X : Inport
  T_c_N : Inport  Port=2
  alpha : Inport  Port=3
  MatrixMultiply3 : Product  Multiplication=Matrix(*)
  Mux : Mux  Inputs=3
  Subsystem1 : Subsystem
  Subsystem2 : Subsystem  Commented=on
  TH : Selector  InputPortWidth=12  IndexOptions=Index vector (dialog)  Indices=[4 5 6]  OutputSizes=1
  Terminator : Terminator
  Transpose1 : Math  Operator=transpose  SaturateOnIntegerOverflow=on
  X-to-wD_N_inC : MATLAB Function  TreatAsAtomicUnit=on
  calc-M : MATLAB Function  TreatAsAtomicUnit=on
  dTHdt : Selector  InputPortWidth=12  IndexOptions=Index vector (dialog)  Indices=[10 11 12]  OutputSizes=1
  dXdt : Selector  InputPortWidth=12  IndexOptions=Index vector (dialog)  Indices=[7 8 9]  OutputSizes=1
  p,q,r : Scope
  q-inf : Subsystem
  M : Outport
  wires:
  MatrixMultiply3/1 -> calc-M/3(wD_N_inN)
  X-to-wD_N_inC/1(wD_N_inC) -> MatrixMultiply3/2
  Transpose1/1 -> MatrixMultiply3/1
  dTHdt/1 -> X-to-wD_N_inC/2(dTHdt)
  TH/1 -> X-to-wD_N_inC/1(TH)
  Mux/1 -> p,q,r/1
  dXdt/1 -> calc-M/1(vel)
  calc-M/4(r) -> Mux/3  "r"
  calc-M/3(q) -> Mux/2  "q"
  calc-M/2(p) -> Mux/1  "p"
  q-inf/1(q-inf-S) -> Terminator/1
  Subsystem1/1(CM) -> calc-M/5(CMpitch)
  q-inf/2(q-inf-S-d) -> calc-M/4(q_inf_times_Sd)
  X/1 -> q-inf/1(X), dXdt/1, dTHdt/1, TH/1
  T_c_N/1 -> calc-M/2(T_c_N), Transpose1/1
  calc-M/1(M) -> M/1  "M"
  alpha/1 -> Subsystem1/1(alpha3)

== system flatball_6dof_plnt_lib/flatball-6dof-HandH/calc-F-M/calc-alpha ==
  X : Inport
  T_c_N : Inport  Port=2
  Dot Product : DotProduct  InputSameDT=on  OutDataTypeStr=Inherit: Inherit via internal rule
  MatrixMultiply3 : Product
  Scope : Scope
  Sum : Sum  Inputs=+-
  calc-alpha : MATLAB Function  TreatAsAtomicUnit=on
  calc-alpha1 : MATLAB Function  TreatAsAtomicUnit=on
  dXdt : Selector  InputPortWidth=12  IndexOptions=Index vector (dialog)  Indices=[7 8 9]  OutputSizes=1
  alpha : Outport
  wires:
  calc-alpha1/1(T_c_Npsi) -> Dot Product/2, MatrixMultiply3/2
  Sum/1 -> Scope/1
  MatrixMultiply3/1 -> Sum/2
  Dot Product/1 -> MatrixMultiply3/1
  dXdt/1 -> calc-alpha/1(dXdt), Sum/1, Dot Product/1
  T_c_N/1 -> calc-alpha/2(T_c_N), calc-alpha1/1(T_c_N)
  X/1 -> dXdt/1
  calc-alpha/1(alpha) -> alpha/1  "alpha"

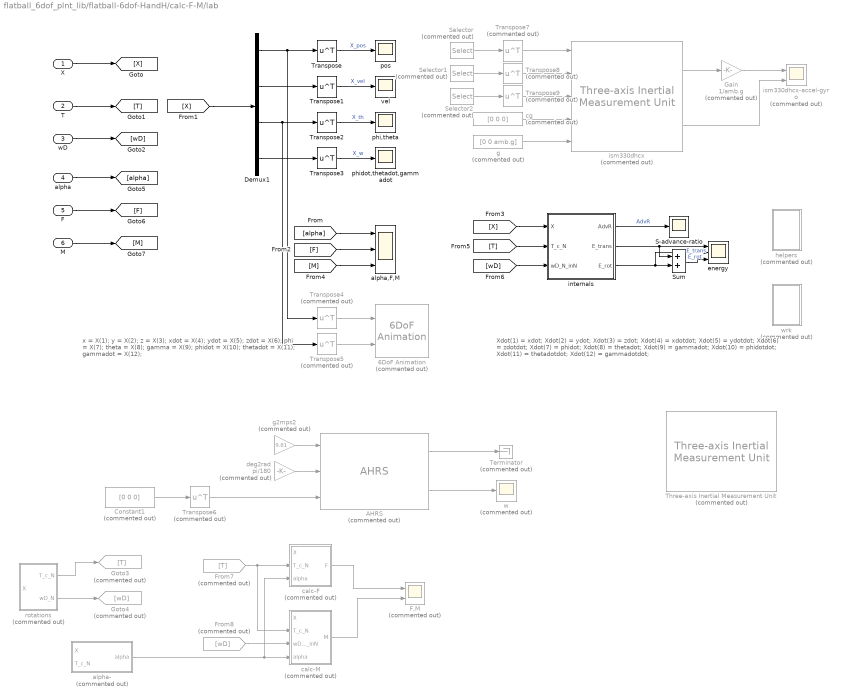
== system flatball_6dof_plnt_lib/flatball-6dof-HandH/calc-F-M/lab ==
  note: Xdot(1) = xdot; Xdot(2) = ydot; Xdot(3) = zdot;
      | Xdot(4) = xdotdot; Xdot(5) = ydotdot; Xdot(6) = zdotdot;
      |
      | Xdot(7) = phidot; Xdot(8) = thetadot; Xdot(9) = gammadot;
      | Xdot(10) = phidotdot; Xdot(11) = thetadotdot; Xdot(12) = gammadotdot;
  note: x = X(1); y = X(2); z = X(3);
      | xdot = X(4); ydot = X(5); zdot = X(6);
      |
      | phi = X(7); theta = X(8); gamma = X(9);
      | phidot = X(10); thetadot = X(11); gammadot = X(12);
  X : Inport
  T : Inport  Port=2
  wD : Inport  Port=3
  alpha : Inport  Port=4
  F : Inport  Port=5
  M : Inport  Port=6
  6DoF Animation : aerolibanim/6DoF Animation  Commented=on  u1=[-20 50 -20 50 -20 5]  u2=0.1  u3=1.0  u4=[-1 -1 -1]  u5=Fixed position  u6=[-200 -20 -10]  u7=10  u8=on
  AHRS : mspfiltlib/AHRS  Commented=on
      settings: SourceProductBaseCode=TF,NV
  Constant1 : Constant  Commented=on  Value=[0 0 0]
  Demux1 : Demux  Outputs=[3 3 3 3]
  F,M : Scope  Commented=on  NumInputPorts=2
  From7 : From  Commented=on  GotoTag=T
  From8 : From  Commented=on  GotoTag=wD
  Gain : Gain  Commented=on  Gain=1/amb.g
  Goto3 : Goto  Commented=on  GotoTag=T
  Goto4 : Goto  Commented=on  GotoTag=wD
  S-advance-ratio : Scope
  Selector : Selector  Commented=on  InputPortWidth=12  IndexOptions=Index vector (dialog)  Indices=[4 5 6]  OutputSizes=1
  Selector1 : Selector  Commented=on  InputPortWidth=12  IndexOptions=Index vector (dialog)  Indices=[7 8 9]  OutputSizes=1
  Selector2 : Selector  Commented=on  InputPortWidth=12  IndexOptions=Index vector (dialog)  Indices=[7 8 9]  OutputSizes=1
  Sum : Sum  Inputs=2
  Terminator : Terminator  Commented=on
  Three-axis Inertial Measurement Unit : aerolibnav/Three-axis Inertial Measurement Unit  Commented=on  units=Metric (MKS)  imu=[0 0 0]  i_Ts=0  dtype_a=on  w_a=190  z_a=0.707  a_sf_cc=[1 0 0; 0 1 0; 0 0 1]  a_bias=[0 0 0]  a_sat="[-inf  -inf  -inf  inf inf inf]"  dtype_g=on  w_g=190  z_g=0.707  g_sf_cc=[1 0 0; 0 1 0; 0 0 1]  g_bias=[0 0 0]  g_sens=[0 0 0]  g_sat="[-inf  -inf  -inf  inf inf inf]"  i_rand=on  i_seeds=[23093 23094 23095 23096 23097 23098]  i_pow=[0.001 0.001 0.001 0.0001 0.0001 0.0001]
  Transpose{,1..3} (4 alike) : Math  Operator=transpose  SaturateOnIntegerOverflow=on
  Transpose{4..9} (6 alike) : Math  Commented=on  Operator=transpose  SaturateOnIntegerOverflow=on
  alpha,F,M : Scope  NumInputPorts=3
  alpha- : MATLAB Function  Commented=on  TreatAsAtomicUnit=on
  calc-F : Subsystem  Commented=on
  calc-M : Subsystem  Commented=on
  cg : Constant  Commented=on  Value=[0 0 0]
  deg2rad : Gain  Commented=on  Gain=pi/180
  energy : Scope  NumInputPorts=3
  g : Constant  Commented=on  Value=[0 0 amb.g]
  g2mps2 : Gain  Commented=on  Gain=9.81
  helpers : Subsystem  Commented=on
  internals : MATLAB Function  TreatAsAtomicUnit=on
  ism330dhcx : aerolibnav/Three-axis Inertial Measurement Unit  Commented=on  units=Metric (MKS)  imu=[-2e-3 1e-3 -5e-3]  i_Ts=0  dtype_a=on  w_a=190  z_a=0.707  a_sf_cc=[1 0 0; 0 1 0; 0 0 1]  a_bias=[0 0 0]  a_sat="[-inf  -inf  -inf  inf inf inf]"  dtype_g=on  w_g=190  z_g=0.707  g_sf_cc=[1 0 0; 0 1 0; 0 0 1]  g_bias=[0 0 0]  g_sens=[0 0 0]  g_sat="[-inf  -inf  -inf  inf inf inf]"  i_rand=on  i_seeds=[23093 23094 23095 23096 23097 23098]  i_pow=[0.001 0.001 0.001 0.0001 0.0001 0.0001]
  ism330dhcx-accel-gyro : Scope  Commented=on  NumInputPorts=2
  phi,theta : Scope
  phidot,thetadot,gammadot : Scope
  pos : Scope
  rotations : Subsystem  Commented=on
  vel : Scope
  w : Scope  Commented=on
  wrk : Subsystem  Commented=on
  wires:
  ism330dhcx/2 -> ism330dhcx-accel-gyro/2
  Gain/1 -> ism330dhcx-accel-gyro/1
  Selector2/1 -> Transpose9/1
  Selector1/1 -> Transpose8/1
  Transpose9/1 -> ism330dhcx/3
  ism330dhcx/1 -> Gain/1
  cg/1 -> ism330dhcx/4
  Transpose8/1 -> ism330dhcx/2
  g/1 -> ism330dhcx/5
  Selector/1 -> Transpose7/1
  Transpose7/1 -> ism330dhcx/1
  AHRS/1 -> Terminator/1
  deg2rad/1 -> AHRS/2
  g2mps2/1 -> AHRS/1
  AHRS/2 -> w/1
  Constant1/1 -> Transpose6/1
  Transpose6/1 -> AHRS/3
  Transpose5/1 -> 6DoF Animation/2
  Transpose4/1 -> 6DoF Animation/1
  Transpose3/1 -> phidot,thetadot,gammadot/1  "X_w"
  Transpose2/1 -> phi,theta/1  "X_th"
  Transpose1/1 -> vel/1  "X_vel"
  Transpose/1 -> pos/1  "X_pos"
  [M] -> alpha,F,M/3
  [F] -> alpha,F,M/2
  [alpha] -> alpha,F,M/1
  M/1 -> [M]
  alpha/1 -> [alpha]
  F/1 -> [F]
  wD/1 -> [wD]
  T/1 -> [T]
  X/1 -> [X]
  [X] -> Demux1/1
  Demux1/2 -> Transpose1/1
  Demux1/1 -> Transpose/1, Transpose4/1
  Demux1/3 -> Transpose2/1, Transpose5/1
  Demux1/4 -> Transpose3/1
  internals/2(E_trans) -> energy/1, Sum/1  "E_trans"
  [X] -> internals/1(X)
  Sum/1 -> energy/3
  [T] -> internals/2(T_c_N)
  internals/1(AdvR) -> S-advance-ratio/1  "AdvR"
  [wD] -> internals/3(wD_N_inN)
  internals/3(E_rot) -> energy/2, Sum/2  "E_rot"
  rotations/2(wD_N) -> Goto4/1
  rotations/1(T_c_N) -> Goto3/1
  calc-F/1(F) -> F,M/1
  calc-M/1(M) -> F,M/2
  From8/1 -> calc-M/3(wD_N_inN)
  alpha-/1(alpha) -> calc-M/4(alpha), calc-F/3(alpha)
  From7/1 -> calc-F/2(T_c_N), calc-M/2(T_c_N)

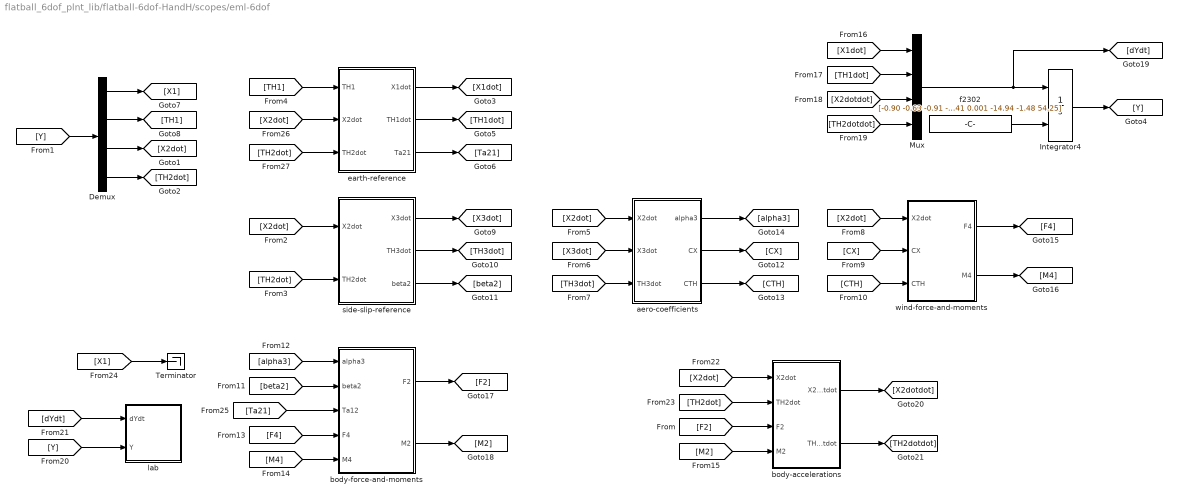
== system flatball_6dof_plnt_lib/flatball-6dof-HandH/scopes/eml-6dof ==
  Demux : Demux  Outputs=[3 3 3 3]
  Integrator4 : Integrator  InitialConditionSource=external
  Mux : Mux
  Terminator : Terminator
  aero-coefficients : MATLAB Function  TreatAsAtomicUnit=on
  body-accelerations : MATLAB Function  TreatAsAtomicUnit=on
  body-force-and-moments : MATLAB Function  TreatAsAtomicUnit=on
  earth-reference : MATLAB Function  TreatAsAtomicUnit=on
  f2302 : Constant  Value=[-0.90 -0.63 -0.91 -0.07 0.21 5.03 13.42 -0.41 0.001 -14.94 -1.48 54.25]
  lab : Subsystem
  side-slip-reference : MATLAB Function  TreatAsAtomicUnit=on
  wind-force-and-moments : MATLAB Function  TreatAsAtomicUnit=on
  wires:
  earth-reference/1(X1dot) -> [X1dot]
  earth-reference/2(TH1dot) -> [TH1dot]
  earth-reference/3(Ta21) -> [Ta21]
  [Y] -> Demux/1
  Demux/1 -> [X1]
  Demux/2 -> [TH1]
  Demux/3 -> [X2dot]
  Demux/4 -> [TH2dot]
  [X2dot] -> side-slip-reference/1(X2dot)
  [TH2dot] -> side-slip-reference/2(TH2dot)
  side-slip-reference/1(X3dot) -> [X3dot]
  side-slip-reference/2(TH3dot) -> [TH3dot]
  side-slip-reference/3(beta2) -> [beta2]
  [TH1] -> earth-reference/1(TH1)
  [X2dot] -> aero-coefficients/1(X2dot)
  [X3dot] -> aero-coefficients/2(X3dot)
  [TH3dot] -> aero-coefficients/3(TH3dot)
  aero-coefficients/3(CTH) -> [CTH]
  aero-coefficients/2(CX) -> [CX]
  aero-coefficients/1(alpha3) -> [alpha3]
  [X2dot] -> wind-force-and-moments/1(X2dot)
  [CX] -> wind-force-and-moments/2(CX)
  [CTH] -> wind-force-and-moments/3(CTH)
  [beta2] -> body-force-and-moments/2(beta2)
  [alpha3] -> body-force-and-moments/1(alpha3)
  wind-force-and-moments/1(F4) -> [F4]
  wind-force-and-moments/2(M4) -> [M4]
  [F4] -> body-force-and-moments/4(F4)
  [M4] -> body-force-and-moments/5(M4)
  body-force-and-moments/1(F2) -> [F2]
  body-force-and-moments/2(M2) -> [M2]
  [TH2dotdot] -> Mux/4
  Mux/1 -> Integrator4/1, [dYdt]
  [TH1dot] -> Mux/2
  [X1dot] -> Mux/1
  f2302/1 -> Integrator4/2
  [X2dotdot] -> Mux/3
  Integrator4/1 -> [Y]
  [dYdt] -> lab/1(dYdt)
  [Y] -> lab/2(Y)
  [F2] -> body-accelerations/3(F2)
  [M2] -> body-accelerations/4(M2)
  [X2dot] -> body-accelerations/1(X2dot)
  [TH2dot] -> body-accelerations/2(TH2dot)
  body-accelerations/2(TH2dotdot) -> [TH2dotdot]
  body-accelerations/1(X2dotdot) -> [X2dotdot]
  [Ta21] -> body-force-and-moments/3(Ta12)
  [X1] -> Terminator/1
  [X2dot] -> earth-reference/2(X2dot)
  [TH2dot] -> earth-reference/3(TH2dot)

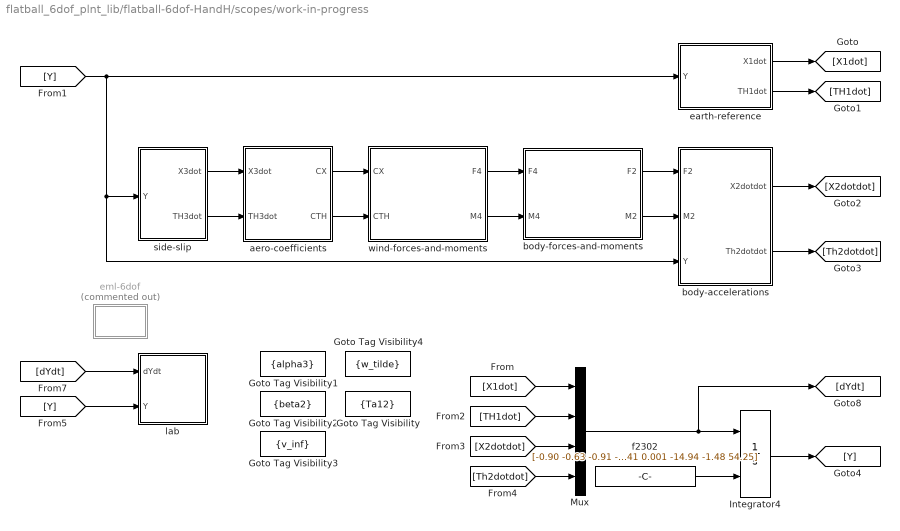
== system flatball_6dof_plnt_lib/flatball-6dof-HandH/scopes/work-in-progress ==
  Goto Tag Visibility : GotoTagVisibility  GotoTag=Ta12
  Goto Tag Visibility1 : GotoTagVisibility  GotoTag=alpha3
  Goto Tag Visibility2 : GotoTagVisibility  GotoTag=beta2
  Goto Tag Visibility3 : GotoTagVisibility  GotoTag=v_inf
  Goto Tag Visibility4 : GotoTagVisibility  GotoTag=w_tilde
  Integrator4 : Integrator  InitialConditionSource=external
  Mux : Mux
  aero-coefficients : Subsystem
  body-accelerations : Subsystem
  body-forces-and-moments : Subsystem
  earth-reference : Subsystem
  eml-6dof : Subsystem  Commented=on
  f2302 : Constant  Value=[-0.90 -0.63 -0.91 -0.07 0.21 5.03 13.42 -0.41 0.001 -14.94 -1.48 54.25]
  lab : Subsystem
  side-slip : Subsystem
  wind-forces-and-moments : Subsystem
  wires:
  [X1dot] -> Mux/1
  [Y] -> lab/2(Y)
  [X2dotdot] -> Mux/3
  [Th2dotdot] -> Mux/4
  [dYdt] -> lab/1(dYdt)
  [TH1dot] -> Mux/2
  body-accelerations/1(X2dotdot) -> [X2dotdot]
  Mux/1 -> [dYdt], Integrator4/1
  Integrator4/1 -> [Y]
  [Y] -> earth-reference/1(Y), side-slip/1(Y), body-accelerations/3(Y)
  f2302/1 -> Integrator4/2
  body-accelerations/2(Th2dotdot) -> [Th2dotdot]
  earth-reference/2(TH1dot) -> [TH1dot]
  earth-reference/1(X1dot) -> [X1dot]
  body-forces-and-moments/2(M2) -> body-accelerations/2(M2)
  wind-forces-and-moments/2(M4) -> body-forces-and-moments/2(M4)
  wind-forces-and-moments/1(F4) -> body-forces-and-moments/1(F4)
  side-slip/2(TH3dot) -> aero-coefficients/2(TH3dot)
  body-forces-and-moments/1(F2) -> body-accelerations/1(F2)
  aero-coefficients/1(CX) -> wind-forces-and-moments/1(CX)
  side-slip/1(X3dot) -> aero-coefficients/1(X3dot)
  aero-coefficients/2(CTH) -> wind-forces-and-moments/2(CTH)

== system flatball_6dof_plnt_lib/flatball-6dof-HandH/calc-F-M/calc-F/aero-coeff ==
  alpha : Inport
  Subsystem : Subsystem
  Subsystem1 : Subsystem
  calc-Cd : Subsystem  Commented=on
  calc-Cl : Subsystem  Commented=on
  Cl : Outport
  Cd : Outport  Port=2
  wires:
  Subsystem/1(Cdrag) -> Cd/1  "Cdrag"
  Subsystem1/1(Clift) -> Cl/1  "Clift"
  alpha/1 -> Subsystem/1(alpha3), Subsystem1/1(alpha3)

== system flatball_6dof_plnt_lib/flatball-6dof-HandH/calc-F-M/calc-F/q-inf ==
  X : Inport
  Gain : Gain  Gain=0.5
  Product1 : Product  Inputs=3
  Product2 : Product
  S : Constant  Value=disc.A
  Square : Math  Operator=square  SaturateOnIntegerOverflow=on
  d : Constant  Value=disc.d
  dXdt : Selector  InputPortWidth=12  IndexOptions=Index vector (dialog)  Indices=[7 8 9]  OutputSizes=1
  rho : Constant  Value=amb.rho
  vector-norm : MATLAB Function  TreatAsAtomicUnit=on
  q-inf-S : Outport
  q-inf-S-d : Outport  Port=2
  wires:
  dXdt/1 -> vector-norm/1(vec)
  d/1 -> Product2/2
  Product2/1 -> q-inf-S-d/1
  X/1 -> dXdt/1
  Gain/1 -> q-inf-S/1, Product2/1
  Square/1 -> Product1/1
  S/1 -> Product1/2
  vector-norm/1(norm) -> Square/1
  rho/1 -> Product1/3
  Product1/1 -> Gain/1

== system flatball_6dof_plnt_lib/flatball-6dof-HandH/calc-F-M/calc-M/Subsystem1 ==
  alpha3 : Inport
  1-D Lookup Table : Lookup_n-D  NumberOfTableDimensions=1  BreakpointsForDimension1=disc.aoa_data  Table=disc.CM_data  InterpMethod=Cubic spline  ExtrapMethod=Cubic spline  InternalRulePriority=Speed  RndMeth=Simplest  InputSameDT=on
  Ground : Ground
  Product1 : Product  Inputs=**
  Sum1 : Sum
  Sum2 : Sum
  Terminator : Terminator
  mg : Constant  Value=disc.CM0
  mg1 : Constant  Value=disc.CMa
  CM : Outport
  wires:
  Ground/1 -> Sum1/2
  Sum1/1 -> CM/1
  Sum2/1 -> Terminator/1
  mg/1 -> Sum2/1
  1-D Lookup Table/1 -> Sum1/1
  Product1/1 -> Sum2/2
  alpha3/1 -> Product1/1, 1-D Lookup Table/1
  mg1/1 -> Product1/2

== system flatball_6dof_plnt_lib/flatball-6dof-HandH/calc-F-M/calc-M/Subsystem2 ==
  alpha : Inport
  CM0 : Constant  Value=disc.CM0
  CMa : Constant  Value=disc.CMa
  Product : Product
  Sum1 : Sum
  Cm : Outport
  wires:
  alpha/1 -> Product/2
  CM0/1 -> Sum1/1
  CMa/1 -> Product/1
  Product/1 -> Sum1/2
  Sum1/1 -> Cm/1

== system flatball_6dof_plnt_lib/flatball-6dof-HandH/calc-F-M/calc-M/q-inf ==
  X : Inport
  Gain : Gain  Gain=0.5
  Product1 : Product  Inputs=3
  Product2 : Product
  S : Constant  Value=disc.A
  Square : Math  Operator=square  SaturateOnIntegerOverflow=on
  d : Constant  Value=disc.d
  dXdt : Selector  InputPortWidth=12  IndexOptions=Index vector (dialog)  Indices=[7 8 9]  OutputSizes=1
  rho : Constant  Value=amb.rho
  vector-norm : MATLAB Function  TreatAsAtomicUnit=on
  q-inf-S : Outport
  q-inf-S-d : Outport  Port=2
  wires:
  dXdt/1 -> vector-norm/1(vec)
  Product1/1 -> Gain/1
  rho/1 -> Product1/3
  vector-norm/1(norm) -> Square/1
  S/1 -> Product1/2
  Square/1 -> Product1/1
  Gain/1 -> Product2/1, q-inf-S/1
  X/1 -> dXdt/1
  Product2/1 -> q-inf-S-d/1
  d/1 -> Product2/2

== system flatball_6dof_plnt_lib/flatball-6dof-HandH/calc-F-M/lab/calc-F ==
  X : Inport
  T_c_N : Inport  Port=2
  alpha : Inport  Port=3
  Fg_N : Constant  Value=[0 0 disc.m*amb.g]'
  Terminator : Terminator
  X-to-vel : MATLAB Function  TreatAsAtomicUnit=on
  aero-coeff : Subsystem
  calc-F : MATLAB Function  TreatAsAtomicUnit=on
  q-inf : Subsystem
  F : Outport
  wires:
  q-inf/2(q-inf-S-d) -> Terminator/1
  aero-coeff/2(Cd) -> calc-F/5(CDrag)
  aero-coeff/1(Cl) -> calc-F/4(CLift)
  alpha/1 -> aero-coeff/1(alpha)
  q-inf/1(q-inf-S) -> calc-F/6(q_inf_times_S)
  calc-F/1(F) -> F/1
  Fg_N/1 -> calc-F/3(Fg_N)
  T_c_N/1 -> calc-F/2(T_c_N)
  X/1 -> X-to-vel/1(X), q-inf/1(X)
  X-to-vel/1(vel) -> calc-F/1(vel)

== system flatball_6dof_plnt_lib/flatball-6dof-HandH/calc-F-M/lab/calc-M ==
  X : Inport
  T_c_N : Inport  Port=2
  wD_N_inN : Inport  Port=3
  alpha : Inport  Port=4
  Terminator : Terminator
  X-to-vel : MATLAB Function  TreatAsAtomicUnit=on
  aero-coeff : Subsystem
  calc-M : MATLAB Function  TreatAsAtomicUnit=on
  q-inf : Subsystem
  M : Outport
  wires:
  q-inf/1(q-inf-S) -> Terminator/1
  wD_N_inN/1 -> calc-M/3(wD_N_inN)
  aero-coeff/1(Cm) -> calc-M/4(CMpitch)
  q-inf/2(q-inf-S-d) -> calc-M/5(q_inf_times_Sd)
  X-to-vel/1(vel) -> calc-M/1(vel)
  X/1 -> q-inf/1(X), X-to-vel/1(X)
  T_c_N/1 -> calc-M/2(T_c_N)
  calc-M/1(M) -> M/1
  alpha/1 -> aero-coeff/1(alpha)

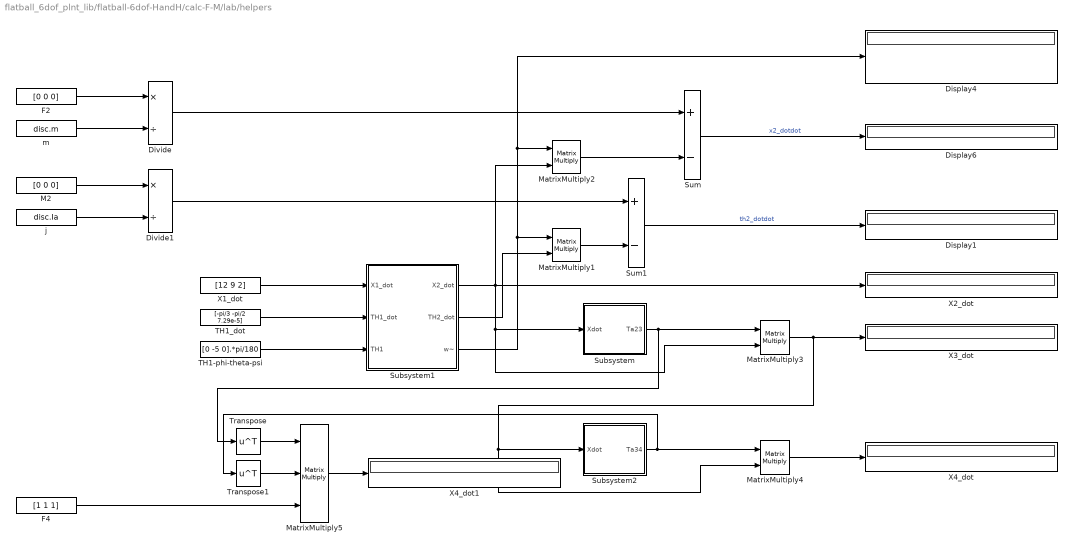
== system flatball_6dof_plnt_lib/flatball-6dof-HandH/calc-F-M/lab/helpers ==
  Display1 : Display
  Display4 : Display
  Display6 : Display
  Divide : Product  Inputs=*/
  Divide1 : Product  Inputs=*/
  F2 : Constant  Value=[0 0 0]
  F4 : Constant  Value=[1 1 1]
  M2 : Constant  Value=[0 0 0]
  MatrixMultiply{1..4} (4 alike) : Product  Multiplication=Matrix(*)
  MatrixMultiply5 : Product  Inputs=***  Multiplication=Matrix(*)
  Subsystem : Subsystem
  Subsystem1 : Subsystem
  Subsystem2 : Subsystem
  Sum : Sum  Inputs=+-
  Sum1 : Sum  Inputs=+-
  TH1-phi-theta-psi : Constant  Value=[0 -5 0].*pi/180
  TH1_dot : Constant  Value=[-pi/3 -pi/2 7.29e-5]
  Transpose : Math  Operator=transpose  SaturateOnIntegerOverflow=on
  Transpose1 : Math  Operator=transpose  SaturateOnIntegerOverflow=on
  X1_dot : Constant  Value=[12 9 2]
  X2_dot : Display
  X3_dot : Display
  X4_dot : Display
  X4_dot1 : Display
  j : Constant  Value=disc.Ia
  m : Constant  Value=disc.m
  wires:
  MatrixMultiply5/1 -> X4_dot1/1
  F4/1 -> MatrixMultiply5/3
  Transpose/1 -> MatrixMultiply5/1
  Transpose1/1 -> MatrixMultiply5/2
  MatrixMultiply4/1 -> X4_dot/1
  Subsystem2/1(Ta34) -> MatrixMultiply4/1, Transpose1/1
  MatrixMultiply3/1 -> X3_dot/1, Subsystem2/1(Xdot), MatrixMultiply4/2
  Subsystem/1(Ta23) -> MatrixMultiply3/1, Transpose/1
  Sum1/1 -> Display1/1  "th2_dotdot"
  Subsystem1/2(TH2_dot) -> MatrixMultiply1/2
  MatrixMultiply1/1 -> Sum1/2
  Divide1/1 -> Sum1/1
  M2/1 -> Divide1/1
  j/1 -> Divide1/2
  Sum/1 -> Display6/1  "x2_dotdot"
  Divide/1 -> Sum/1
  m/1 -> Divide/2
  F2/1 -> Divide/1
  Subsystem1/1(X2_dot) -> Subsystem/1(Xdot), MatrixMultiply3/2, X2_dot/1, MatrixMultiply2/2
  Subsystem1/3(w~) -> MatrixMultiply2/1, Display4/1, MatrixMultiply1/1
  MatrixMultiply2/1 -> Sum/2
  TH1-phi-theta-psi/1 -> Subsystem1/3(TH1)
  TH1_dot/1 -> Subsystem1/2(TH1_dot)
  X1_dot/1 -> Subsystem1/1(X1_dot)

== system flatball_6dof_plnt_lib/flatball-6dof-HandH/calc-F-M/lab/rotations ==
  X : Inport
  MatrixMultiply3 : Product  Multiplication=Matrix(*)
  Transpose : Math  Operator=transpose  SaturateOnIntegerOverflow=on
  Transpose1 : Math  Operator=transpose  SaturateOnIntegerOverflow=on
  X-to-T_c_N : MATLAB Function  TreatAsAtomicUnit=on
  X-to-wD_N_inC : MATLAB Function  TreatAsAtomicUnit=on
  T_c_N : Outport
  wD_N : Outport  Port=2
  wires:
  X/1 -> X-to-T_c_N/1(X), X-to-wD_N_inC/1(X)
  MatrixMultiply3/1 -> wD_N/1
  Transpose/1 -> MatrixMultiply3/2
  X-to-wD_N_inC/1(wD_N_inC) -> Transpose/1
  Transpose1/1 -> MatrixMultiply3/1
  X-to-T_c_N/1(T_c_N) -> T_c_N/1, Transpose1/1

== system flatball_6dof_plnt_lib/flatball-6dof-HandH/calc-F-M/lab/wrk ==
  6DoF Animation : aerolibanim/6DoF Animation  Commented=on  u1=[-10 100 -20 100 -10 10]  u2=0.01  u3=5  u4=[1 0 -5]  u5=Fixed position  u6=[100 50 -500]  u7=10  u8=on
  Demux : Demux  Commented=on  Outputs=[3 3 3 3]
  From : From  Commented=on  GotoTag=x1
  From1 : From  Commented=on  GotoTag=x1dt
  From2 : From  Commented=on  GotoTag=theta1
  From3 : From  Commented=on  GotoTag=theta1dt
  From5 : From  Commented=on  GotoTag=theta1
  From6 : From  Commented=on  GotoTag=theta1dt
  From7 : From  Commented=on  GotoTag=x1dt
  Transpose{3..6} (4 alike) : Math  Commented=on  Operator=transpose  SaturateOnIntegerOverflow=on
  c&p : Subsystem  Commented=on
  flatball_6dof : MATLAB Function  Commented=on  TreatAsAtomicUnit=on
  flatball_6dof_v1p0 : MATLAB Function  Commented=on  TreatAsAtomicUnit=on
  flatball_6dof_v1p1 : MATLAB Function  Commented=on  TreatAsAtomicUnit=on
  hummel : Subsystem  Commented=on
  wires:
  From7/1 -> hummel/1(vel)
  From6/1 -> hummel/3(TH-dt)
  From5/1 -> hummel/2(TH)
  Transpose6/1 -> c&p/4(theta1dt)
  Transpose4/1 -> c&p/2(x1dt)
  Transpose5/1 -> c&p/3(theta1)
  From1/1 -> Transpose4/1
  Demux/1 -> 6DoF Animation/1
  Transpose3/1 -> c&p/1(x1)
  Demux/3 -> 6DoF Animation/2
  From3/1 -> Transpose6/1
  From2/1 -> Transpose5/1
  From/1 -> Transpose3/1
